simulink model "signal"  (Simulink 9.1)
settings: Solver=FixedStepAuto  StartTime=0.0  StopTime=200  FixedStep=0.1  RelTol=1e-3
libraries: simulink x2
settings Model: Creator=Administrator  LastModifiedBy=Administrator
settings DataIOCC: SaveFormat=Dataset
settings OptimizationCC: LifeSpan=auto
settings DebuggingCC: UnderspecifiedInitializationDetection=Simplified  MergeDetectMultiDrivingBlocksExec=error  SFUnexpectedBacktrackingDiag=error  SFNoUnconditionalDefaultTransitionDiag=error  SFExecutionAtInitializationDiag=warning
settings HardwareCC: ProdBitPerPointer=64  ProdBitPerSizeT=64  ProdBitPerPtrDiffT=64  ProdLargestAtomicFloat=Float  ProdIntDivRoundTo=Zero  ProdEndianess=LittleEndian  ProdWordSize=64  ProdHWDeviceType=Intel->x86-64 (Windows64)
settings ModelReferenceCC: PropagateSignalLabelsOutOfModel=on
settings CodeAppCC: StateflowObjectComments=off
settings GRTTargetCC: TargetLangStandard=C99 (ISO)  CombineOutputUpdateFcns=on  GRTInterface=off
settings ConfigComp: CovMetricSettings=dwe  CovHtmlReporting=off  CovSaveCumulativeToWorkspaceVar=off  CovSaveSingleToWorkspaceVar=off  CovExternalEMLEnable=on

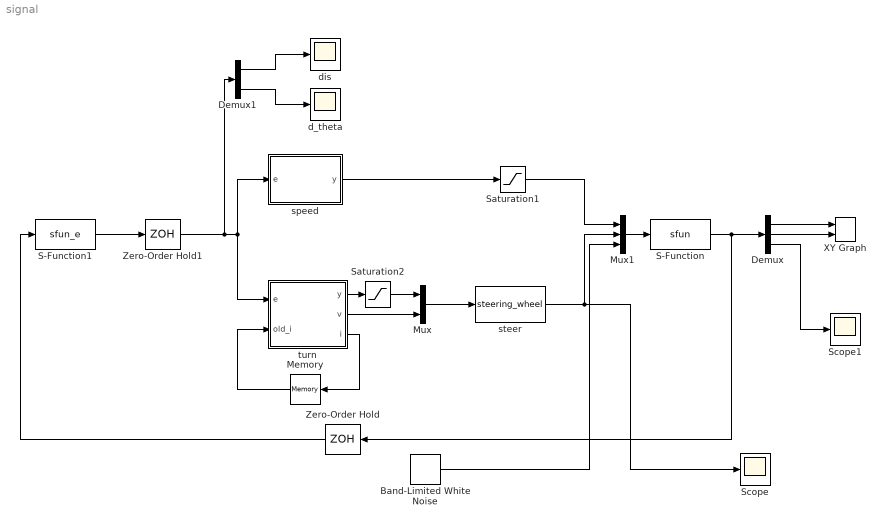
== system signal ==
  Band-Limited White Noise : simulink/Sources/Band-Limited White Noise  Cov=[0.00]  Ts=0.1  seed=[23341]
  Demux : Demux  Outputs=3
  Demux1 : Demux  Outputs=2
  Memory : Memory
  Mux : Mux  Inputs=2
  Mux1 : Mux  Inputs=3
  S-Function : S-Function  FunctionName=sfun  SFunctionDeploymentMode=off  EnableBusSupport=off
  S-Function1 : S-Function  FunctionName=sfun_e  SFunctionDeploymentMode=off  EnableBusSupport=off
  Saturation1 : Saturate  UpperLimit=1  LowerLimit=0
  Saturation2 : Saturate  UpperLimit=pi/3  LowerLimit=-pi/3
  Scope : Scope
  Scope1 : Scope
  XY Graph : simulink/Sinks/XY Graph  xmin=0  xmax=10  ymin=0  ymax=0.5  st=-1
  Zero-Order Hold : ZeroOrderHold  SampleTime=0.1
  Zero-Order Hold1 : ZeroOrderHold  SampleTime=-1
  d_theta : Scope
  dis : Scope
  speed : MATLAB Function  TreatAsAtomicUnit=on
  steer : S-Function  FunctionName=steering_wheel  SFunctionDeploymentMode=off  EnableBusSupport=off
  turn : MATLAB Function  TreatAsAtomicUnit=on
  wires:
  S-Function/1 -> Zero-Order Hold/1, Demux/1
  S-Function1/1 -> Zero-Order Hold1/1
  Mux1/1 -> S-Function/1
  Demux/1 -> XY Graph/1
  Demux/2 -> XY Graph/2
  steer/1 -> Mux1/2, Scope/1
  speed/1(y) -> Saturation1/1
  Saturation1/1 -> Mux1/1
  Demux/3 -> Scope1/1
  Demux1/1 -> dis/1
  Demux1/2 -> d_theta/1
  Band-Limited White Noise/1 -> Mux1/3
  turn/3(i) -> Memory/1
  Memory/1 -> turn/2(old_i)
  Zero-Order Hold/1 -> S-Function1/1
  Zero-Order Hold1/1 -> Demux1/1, speed/1(e), turn/1(e)
  Saturation2/1 -> Mux/1
  turn/2(v) -> Mux/2
  Mux/1 -> steer/1
  turn/1(y) -> Saturation2/1

== matlab function turn ==
  data: e input double; y output double; v output double; old_i input double; i output double
function [y, v, i] = fcn(e,old_i)
% y = atan(1.06 * cos(e(2))^3 * (3 * tan(e(2)) + 3 * e(1)));
i = old_i;
if e(1) < 0.15
    i = i + e(1);
end
if i > 200
    i = 200;
end
if i < -200
    i = -200;
end
y = e(2) + atan(1.3 * (e(1) + 1.06*sin(e(2))) / 1) + 0.03 * i ;
if y > 0
    v = 0.270526034059121;
else
    v = -0.270526034059121;
end

== matlab function speed ==
  data: e input double; y output double
function y = fcn(e)

y = 0.7;
